simulink subsystem "random_bit_source_barker"  (R2024b)
settings: Solver=VariableStepAuto  StartTime=0.0  StopTime=10.0  RelTol=1e-3
undefined symbols (not defined in the file or in its folder): Param
libraries: commrandsrc3 x1, dspsigops x1
settings Model: Creator=rober  LastModifiedBy=rober

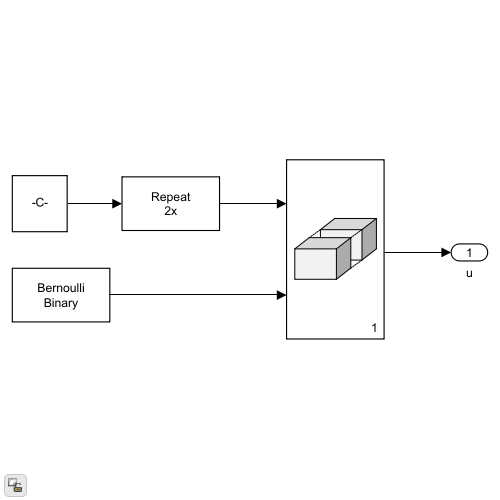
[thumbnail: Simulink's stored preview of the top-level diagram]
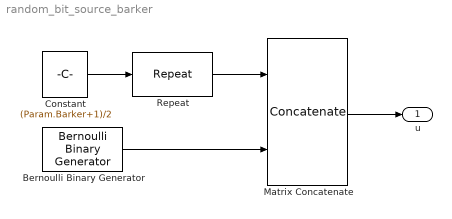
== system random_bit_source_barker ==
  Bernoulli Binary Generator : commrandsrc3/Bernoulli Binary Generator  ProbabilityOfZero=0.5  SeedSource=Auto  Seed=0  SampleTime=1/Param.PayloadLength*Param.FrameTime  SamplesPerFrame=Param.PayloadLength  OutputDataType=double  SimulateUsing=Code generation
  Constant : Constant  Value=(Param.Barker+1)/2  VectorParams1D=off
  Matrix Concatenate : Concatenate  Mode=Multidimensional array
  Repeat : dspsigops/Repeat  FactorSource=Dialog parameter  N=2  Nmax=16  InputProcessing=Columns as channels (frame based)  RateOptions=Enforce single-rate processing  ic=0  mode=Unused parameter value
      settings: LibrarySourceBlock=commsequence2/Repeat
  u : Outport
  wires:
  Bernoulli Binary Generator/1 -> Matrix Concatenate/2
  Matrix Concatenate/1 -> u/1
  Repeat/1 -> Matrix Concatenate/1
  Constant/1 -> Repeat/1
